simulink model "Bebop10_from_exp"  (R2018a)
settings: Solver=VariableStepAuto  StartTime=0.0  StopTime=100  FixedStep=0.0025  MaxStep=1  MinStep=0.005  RelTol=10  AbsTol=10
values from neighbouring files (symbols this model uses):
  flightplan = [dist,0,height,deg2rad(090) ... (first row only)    [compare_cubic_spline_1.m]    (also in initialize_race_realtime.m = flightplan - [0.5*min(flightplan(:,1:2))+0.5*max(flightplan(; initialize_race_realtime_backup_cubic.m; plot_sim.m = [ 4.348, -0.278, height, deg2rad(  0); test_b_spline.m)
  FOV = 1.05    [initialize_race_realtime_backup_cubic.m]
  g = 9.81    [initialize_race_no_realtime.m]    (also in initialize_race_realtime.m; initialize_race_realtime_backup_cubic.m; moving_average_rls_own.m = P(i-1)*meas*(lambda+meas*P(i-1)*meas)^-1)
  gate_size = 1.4    [initialize_race_realtime.m]    (also in initialize_race_realtime_backup_cubic.m)
  gates = sim_gates(:,:,1)    [eval_sim.m]    (also in initialize_race_realtime.m = flightplan + pert; initialize_race_realtime_backup_cubic.m = [dist,0,height,deg2rad(110); plot_sim.m)
  HFOV = VFOV*resolution(1)/resolution(2)    [initialize_race_realtime.m]
  I = [1 0 0 ... (first row only)    [Bebop_sim_init.m]    (also in initialize_race_no_realtime.m; initialize_race_realtime.m; initialize_race_realtime_backup_cubic.m; moving_averge_rls_download.m = ones(1,N))
  m = 0.68    [calc_plot_spline.m]    (also in calc_spline.m; compare_cubic_spline_1.m = vpasolve(e,r); compare_cubic_spline_2.m = r/3*(-sin(dp)+sqrt(sin(dp)^2-6*cos(dp)+6)); initialize_race_no_realtime.m = 2)
  mass = 2    [Bebop_sim_init.m]    (also in initialize_race_realtime.m = 0.5)
  max_rot_Z = (90)*pi/180    (= 1.57079632679)    [Bebop_sim_init.m]    (also in initialize_race_no_realtime.m = 1.0471975512; initialize_race_realtime.m = 3.14159265359; initialize_race_realtime_backup_cubic.m; run_batch1.m = list_agility(idx_agility)*max_rot_Z)
  max_theta_X = (40)*pi/180    (= 0.698131700798)    [Bebop_sim_init.m]    (also in initialize_race_no_realtime.m = 0.13962634016; initialize_race_realtime.m = 0.418879020479; initialize_race_realtime_backup_cubic.m = 1.308996939; run_batch1.m = list_agility(idx_agility)*max_theta_X)
  max_theta_Y = (40)*pi/180    (= 0.698131700798)    [Bebop_sim_init.m]    (also in initialize_race_no_realtime.m = 0.13962634016; initialize_race_realtime.m = 0.418879020479; initialize_race_realtime_backup_cubic.m = 1.308996939; run_batch1.m = list_agility(idx_agility)*max_theta_Y)
  max_v_Z = .5    (= 0.5)    [Bebop_sim_init.m]    (also in initialize_race_no_realtime.m = 1; initialize_race_realtime.m = 6; initialize_race_realtime_backup_cubic.m = 3; run_batch1.m = list_agility(idx_agility)*max_v_Z)
  max_vel = 2.0    (= 2)    [initialize_race_realtime.m]    (also in initialize_race_realtime_backup_cubic.m = 1.5; run_batch1.m = list_speed(idx_speed); run_batch2.m = list_speed(idx_speed); run_batch3.m = list_speed(idx_speed))
  resolution = 0.5*[1280 720]    [initialize_race_realtime.m]
  spline_init = [P0;P1;P2;P3]    [initialize_race_realtime.m]
  std_dev_eul = 0.25*deg2rad(0.8)*ones(1,3)    [initialize_race_realtime.m]    (also in run_batch1.m = list_sensor_eul(idx_sensor)*dist*ones(1,3); run_batch2.m = list_sensor_eul(idx_sensor)*dist*ones(1,3); run_batch3.m = list_sensor_eul(idx_sensor)*dist*ones(1,3); run_batch4.m = list_sensor_eul(idx_sensor)*dist*ones(1,3))
  std_dev_F = 0.1*max_force*ones(1,3)    [initialize_race_realtime.m]    (also in run_batch1.m = list_actuator(idx_actuator)*max_force*ones(1,3); run_batch2.m = list_actuator(idx_actuator)*max_force*ones(1,3); run_batch3.m = list_actuator(idx_sensor)*max_force*ones(1,3); run_batch4.m = list_actuator(idx_sensor)*max_force*ones(1,3))
  std_dev_M = 0.1*max_moment*[0, 0, 1]    [initialize_race_realtime.m]    (also in run_batch1.m = list_actuator(idx_actuator)*max_moment*[0, 0, 1]; run_batch2.m = list_actuator(idx_actuator)*max_moment*[0, 0, 1]; run_batch3.m = list_actuator(idx_sensor)*max_moment*[0, 0, 1]; run_batch4.m = list_actuator(idx_sensor)*max_moment*[0, 0, 1])
  std_dev_vel = 0.06*ones(1,3)    [initialize_race_realtime.m]    (also in run_batch1.m = list_sensor(idx_sensor)*dist*ones(1,3); run_batch2.m = list_sensor(idx_sensor)*dist*ones(1,3); run_batch3.m = list_sensor(idx_sensor)*dist*ones(1,3); run_batch4.m = list_sensor(idx_sensor)*dist*ones(1,3))
  std_dev_xyz = 0.06*ones(1,3)    [initialize_race_realtime.m]    (also in run_batch1.m = list_sensor(idx_sensor)*dist*ones(1,3); run_batch2.m = list_sensor(idx_sensor)*dist*ones(1,3); run_batch3.m = list_sensor(idx_sensor)*dist*ones(1,3); run_batch4.m = list_sensor(idx_sensor)*dist*ones(1,3))
  two_std_dev_init = [1,1,0.5,deg2rad(30)]    [initialize_race_realtime.m]
  two_std_dev_thres = 0.3    [initialize_race_realtime.m]
  VFOV = 1.05    [initialize_race_realtime.m]
undefined symbols (not defined in the file or in its folder): gray, Rec, SDTV
libraries: sharedtransform x13, visiontextngfix x5, aerolibactuator x4, simulink x3, aerolibutil x2, visionconversions x2, shared6dof x1, vrlib x1, visionanalysis x1, visionstatistics x1, visiontransforms x1
(part 1 of 3)
settings Model: Creator=vinni  LastModifiedBy=lenny
settings SolverCC: MaxConsecutiveMinStep=99999  ShapePreserveControl=EnableAll  ZeroCrossAlgorithm=Adaptive
settings DebuggingCC: RTPrefix=warning  StringTruncationChecking=warning  WriteAfterWriteMsg=EnableAllAsError  MaxConsecutiveZCsMsg=warning  MultiTaskDSMMsg=warning  MultiTaskCondExecSysMsg=warning  MultiTaskRateTransMsg=warning  ParameterDowncastMsg=warning  ParameterOverflowMsg=warning  ParameterUnderflowMsg=warning  InvalidFcnCallConnMsg=warning  FcnCallInpInsideContextMsg=warning  UniqueDataStoreMsg=warning  ModelReferenceExtraNoncontSigs=warning  NonBusSignalsTreatedAsBus=error
settings HardwareCC: ProdBitPerLong=64  ProdHWDeviceType=Intel->x86-64 (Linux 64)

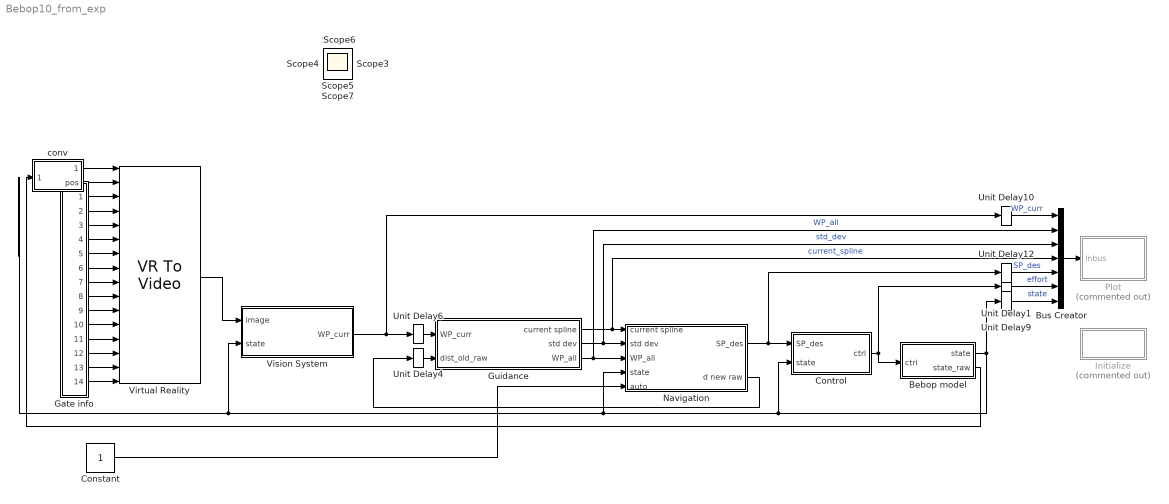
== system Bebop10_from_exp ==
  Bebop model : Subsystem
  Bus Creator : BusCreator  Inputs=7  OutDataTypeStr=Bus: PlotBus  NonVirtualBus=on
  Constant : Constant
  Control : Subsystem
  Gate info : Subsystem
  Guidance : Subsystem
  Initialize : Subsystem  Commented=on  TreatAsAtomicUnit=on
  Navigation : Subsystem
  Plot : MATLAB Function  Commented=on  TreatAsAtomicUnit=on
  Unit Delay{1,4,6,9..10,12} (6 alike) : UnitDelay  SampleTime=-1
  Virtual Reality : vrlib/VR To Video  InstantiateOnLoad=on  SampleTime=0.200  ViewEnable=on  RemoteChange=off  RemoteView=off  FieldsWritten=drone.orientation.4.1.1.double#drone.position.3.1.1.double#G1.rotation.4.1.1.double#G1.translation.3.1.1.double#G2.rotation.4.1.1.double#G2.translation.3.1.1.double#G3.rotation.4.1.1.double#G3.translation.3.1.1.double#G4.rotation.4.1.1.double#G4.translation.3.1.1.double#G5.rotation.4.1.1.double#G5.translation.3.1.1.double#G6.rotation.4.1.1.double#G6.translation.3.1.1.double#G7.rotation.4.1.1.double#G7.translation.3.1.1.double  WorldFileName=race_course.wrl  AutoView=off  VideoDimensions=0.5*[720 1280]  AllowVariableSize=off  FigureProperties="{'Position', 'Name', 'Viewpoint', 'CameraBound', 'CameraDirection', 'CameraPosition', 'CameraUpVector', 'ZoomFactor', 'Antialiasing', 'Headlight', 'Lighting', 'NavPanel', 'Sound', 'StatusBar', 'Stereo3D', 'Stereo3DCameraOffset', 'Stereo3DHIT', 'ToolBar', 'Textures', 'Transparency', 'Triad', 'Wireframe', 'NavZones', 'NavMode', 'NavSpeed', 'CaptureFileFormat', 'CaptureFileName', 'Record2DCompressMethod', 'Record2DCompressQuality', 'Record2D', 'Record2DFileName', 'Record2DFPS'; [3.0000000000000000e+01   6.0000000000000000e+01   6.4000000000000000e+02   3.6000000000000000e+02], '', '_untitled_1', 'on', [0.0000000000000000e+00   0.0000000000000000e+00  -1.0000000000000000e+00], [0.0000000000000000e+00   0.0000000000000000e+00   0.0000000000000000e+00], [0.0000000000000000e+00   1.0000000000000000e+00   0.0000000000000000e+00], [1.0000000000000000e+00], 'off', 'on', 'on', 'none', 'on', 'off', 'off', [1.0000000149011612e-01], [0.0000000000000000e+00], 'off', 'on', 'on', 'none', 'off', 'off', 'fly', 'normal', 'tif', '%f_anim_%n.tif', 'auto', [7.5000000000000000e+01], 'off', '***video***', 'auto'}"
      settings: SourceProductName=Simulink 3D Animation  SourceProductBaseCode=VR
  Vision System : Subsystem
  conv : Subsystem
  Scope{,1..7} (8 alike) : Scope
  wires:
  Vision System/1(WP_curr) -> Unit Delay10/1, Unit Delay6/1
  Control/1(ctrl) -> Bebop model/1(ctrl), Unit Delay1/1
  Unit Delay6/1 -> Guidance/1(WP_curr)
  Unit Delay4/1 -> Guidance/2(dist_old_raw)
  Navigation/1(SP_des) -> Unit Delay12/1, Control/1(SP_des)
  Navigation/2(d new raw) -> Unit Delay4/1
  Bus Creator/1 -> Plot/1(inbus)
  Guidance/3(WP_all) -> Navigation/3(WP_all), Bus Creator/2  "WP_all"
  Guidance/2(std dev) -> Navigation/2(std dev), Bus Creator/3  "std_dev"
  Unit Delay9/1 -> Bus Creator/7  "state"
  Unit Delay10/1 -> Bus Creator/1  "WP_curr"
  Unit Delay12/1 -> Bus Creator/5  "SP_des"
  Guidance/1(current spline) -> Navigation/1(current spline), Bus Creator/4  "current_spline"
  Unit Delay1/1 -> Bus Creator/6  "effort"
  Virtual Reality/1 -> Vision System/1(image)
  Constant/1 -> Navigation/5(auto)
  Bebop model/1(state) -> Control/2(state), Navigation/4(state), Vision System/2(state), Unit Delay9/1
  conv/1(axang) -> Virtual Reality/1
  conv/2(pos) -> Virtual Reality/2
  Gate info/1(O1) -> Virtual Reality/3
  Gate info/2(P1) -> Virtual Reality/4
  Gate info/3(O2) -> Virtual Reality/5
  Gate info/4(P2) -> Virtual Reality/6
  Gate info/5(O3) -> Virtual Reality/7
  Gate info/6(P3) -> Virtual Reality/8
  Gate info/7(O4) -> Virtual Reality/9
  Gate info/8(P4) -> Virtual Reality/10
  Gate info/9(O5) -> Virtual Reality/11
  Gate info/10(P5) -> Virtual Reality/12
  Gate info/11(O6) -> Virtual Reality/13
  Gate info/12(P6) -> Virtual Reality/14
  Gate info/13(O7) -> Virtual Reality/15
  Gate info/14(P7) -> Virtual Reality/16
  Bebop model/2(state_raw) -> conv/1(state)

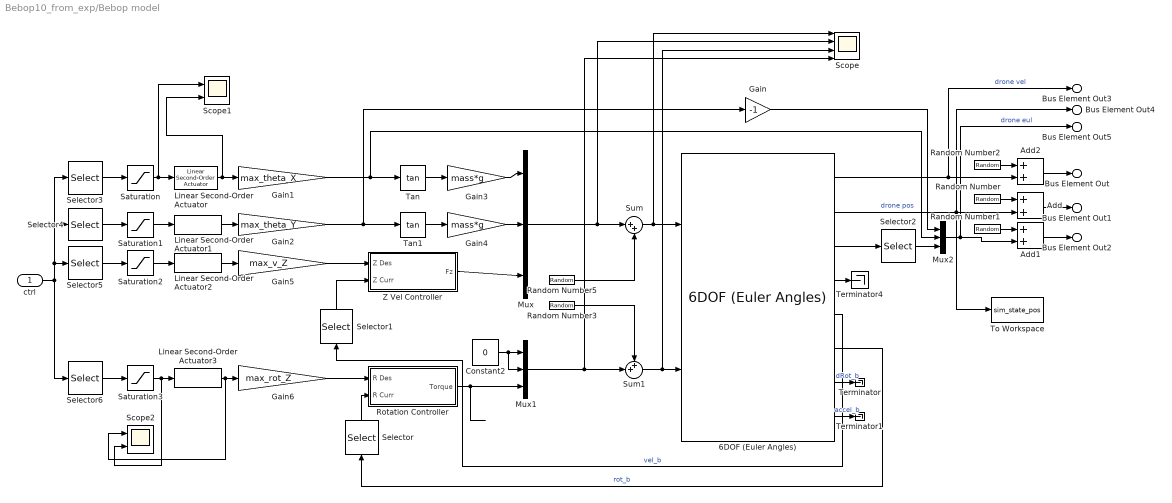
== system Bebop10_from_exp/Bebop model ==
  ctrl : Inport
  6DOF (Euler Angles) : shared6dof/6DOF (Euler Angles)  units=Metric (MKS)  mtype=Fixed  rep=Euler Angles  xme_0=Initial_pos  Vm_0=Initial_vel_b  eul_0=Initial_ori  pm_0=[0 0 0]  mass_0=mass  mass_e=0.5  mass_f=2.0  inertia=I  inertia_e=eye(3)  inertia_f=2*eye(3)  k_quat=1.0  vre_flag=on  abi_flag=off  aMode=0
      settings: SourceProductBaseCode=AE
  Add : Sum
  Add1 : Sum
  Add2 : Sum
  Constant2 : Constant  Value=0
  Gain : Gain  Gain=-1
  Gain1 : Gain  Gain=max_theta_X
  Gain2 : Gain  Gain=max_theta_Y
  Gain3 : Gain  Gain=mass*g
  Gain4 : Gain  Gain=mass*g
  Gain5 : Gain  Gain=max_v_Z
  Gain6 : Gain  Gain=max_rot_Z
  Linear Second-Order Actuator : aerolibactuator/Linear Second-Order Actuator  wn_fin=20  z_fin=3  fin_act_0=0  fin_act_vel=0
      settings: SourceProductName=Aerospace Blockset  SourceProductBaseCode=AE
  Linear Second-Order Actuator1 : aerolibactuator/Linear Second-Order Actuator  wn_fin=20  z_fin=3  fin_act_0=0  fin_act_vel=0
      settings: SourceProductName=Aerospace Blockset  SourceProductBaseCode=AE
  Linear Second-Order Actuator2 : aerolibactuator/Linear Second-Order Actuator  wn_fin=20  z_fin=1  fin_act_0=0  fin_act_vel=0
      settings: SourceProductName=Aerospace Blockset  SourceProductBaseCode=AE
  Linear Second-Order Actuator3 : aerolibactuator/Linear Second-Order Actuator  wn_fin=20  z_fin=1  fin_act_0=0  fin_act_vel=0
      settings: SourceProductName=Aerospace Blockset  SourceProductBaseCode=AE
  Mux : Mux  Inputs=3
  Mux1 : Mux  Inputs=3
  Mux2 : Mux  Inputs=3
  Random Number : RandomNumber  Mean=0*ones(1,3)  Variance=std_dev_xyz.^2.*ones(1,3)  Seed=[4,5,6]  SampleTime=0.1
  Random Number1 : RandomNumber  Mean=0*ones(1,3)  Variance=std_dev_eul.^2.*ones(1,3)  Seed=[7,8,9]  SampleTime=0.1
  Random Number2 : RandomNumber  Mean=0*ones(1,3)  Variance=std_dev_vel.^2.*ones(1,3)  Seed=[1,2,3]  SampleTime=0.1
  Random Number3 : RandomNumber  Mean=0*ones(1,3)  Variance=std_dev_M.^2.*ones(1,3)  Seed=[13,14,15]  SampleTime=0.1
  Random Number5 : RandomNumber  Mean=0*ones(1,3)  Variance=std_dev_F.^2.*ones(1,3)  Seed=[10,11,12]  SampleTime=0.1
  Rotation Controller : Subsystem
  Saturation{,1..3} (4 alike) : Saturate  UpperLimit=1  LowerLimit=-1
  Scope : Scope  NumInputPorts=4
  Scope1 : Scope  NumInputPorts=2
  Scope2 : Scope  NumInputPorts=2
  Selector : Selector  InputPortWidth=3  IndexOptions=Index vector (dialog)  Indices=3  OutputSizes=1
  Selector1 : Selector  InputPortWidth=3  IndexOptions=Index vector (dialog)  Indices=3  OutputSizes=1
  Selector2 : Selector  InputPortWidth=3  IndexOptions=Index vector (dialog)  Indices=3  OutputSizes=1
  Selector3 : Selector  IndexMode=Zero-based  InputPortWidth=4  IndexOptions=Index vector (dialog)  Indices=0  OutputSizes=1
  Selector4 : Selector  IndexMode=Zero-based  InputPortWidth=4  IndexOptions=Index vector (dialog)  Indices=1  OutputSizes=1
  Selector5 : Selector  IndexMode=Zero-based  InputPortWidth=4  IndexOptions=Index vector (dialog)  Indices=2  OutputSizes=1
  Selector6 : Selector  IndexMode=Zero-based  InputPortWidth=4  IndexOptions=Index vector (dialog)  Indices=3  OutputSizes=1
  Sum : Sum  Inputs=|++
  Sum1 : Sum  Inputs=++|
  Tan : Trigonometry  Operator=tan
  Tan1 : Trigonometry  Operator=tan
  Terminator : Terminator
  Terminator1 : Terminator
  Terminator4 : Terminator
  To Workspace : ToWorkspace  VariableName=sim_state_pos  SaveFormat=Timeseries  SampleTime=-1
  Z Vel Controller : Subsystem
  Bus Element Out : Outport  PortName=state  Element=vel
  Bus Element Out1 : Outport  PortName=state  Element=pos
  Bus Element Out2 : Outport  PortName=state  Element=eul
  Bus Element Out3 : Outport  Port=2  PortName=state_raw  Element=vel
  Bus Element Out4 : Outport  Port=2  PortName=state_raw  Element=pos
  Bus Element Out5 : Outport  Port=2  PortName=state_raw  Element=eul
  wires:
  6DOF (Euler Angles)/5 -> Selector1/1  "vel_b"
  Saturation/1 -> Scope1/1, Linear Second-Order Actuator/1
  Tan1/1 -> Gain4/1
  Selector6/1 -> Saturation3/1
  Linear Second-Order Actuator1/1 -> Gain2/1
  Z Vel Controller/1(Fz) -> Mux/3
  6DOF (Euler Angles)/1 -> Bus Element Out3/1, Add2/2  "drone vel"
  Rotation Controller/1(Torque) -> Mux1/3
  Selector/1 -> Rotation Controller/2(R Curr)
  Selector1/1 -> Z Vel Controller/2(Z Curr)
  Gain3/1 -> Mux/1
  Saturation1/1 -> Linear Second-Order Actuator1/1
  6DOF (Euler Angles)/3 -> Selector2/1
  Selector5/1 -> Saturation2/1
  Gain1/1 -> Mux2/2, Tan/1
  Mux/1 -> Scope/2, Sum/1
  Gain5/1 -> Z Vel Controller/1(Z Des)
  Selector4/1 -> Saturation1/1
  Tan/1 -> Gain3/1
  Gain/1 -> Mux2/1
  6DOF (Euler Angles)/4 -> Terminator4/1
  Constant2/1 -> Mux1/2, Mux1/1
  Saturation2/1 -> Linear Second-Order Actuator2/1
  Gain2/1 -> Tan1/1, Gain/1
  Saturation3/1 -> Scope2/2, Linear Second-Order Actuator3/1
  Linear Second-Order Actuator/1 -> Scope1/2, Gain1/1
  Mux1/1 -> Scope/4, Sum1/2
  Gain6/1 -> Rotation Controller/1(R Des)
  Gain4/1 -> Mux/2
  Selector3/1 -> Saturation/1
  6DOF (Euler Angles)/6 -> Selector/1  "rot_b"
  Selector2/1 -> Mux2/3
  6DOF (Euler Angles)/2 -> Bus Element Out4/1, To Workspace/1, Add/2  "drone pos"
  Mux2/1 -> Bus Element Out5/1, Add1/2  "drone eul"
  ctrl/1 -> Selector5/1, Selector4/1, Selector3/1, Selector6/1
  6DOF (Euler Angles)/7 -> Terminator/1  "dRot_b"
  6DOF (Euler Angles)/8 -> Terminator1/1  "accel_b"
  Random Number/1 -> Add/1
  Add/1 -> Bus Element Out1/1
  Random Number2/1 -> Add2/1
  Random Number1/1 -> Add1/1
  Add2/1 -> Bus Element Out/1
  Add1/1 -> Bus Element Out2/1
  Linear Second-Order Actuator2/1 -> Gain5/1
  Linear Second-Order Actuator3/1 -> Scope2/1, Gain6/1
  Sum/1 -> Scope/1, 6DOF (Euler Angles)/1
  Random Number5/1 -> Sum/2
  Random Number3/1 -> Sum1/1
  Sum1/1 -> Scope/3, 6DOF (Euler Angles)/2

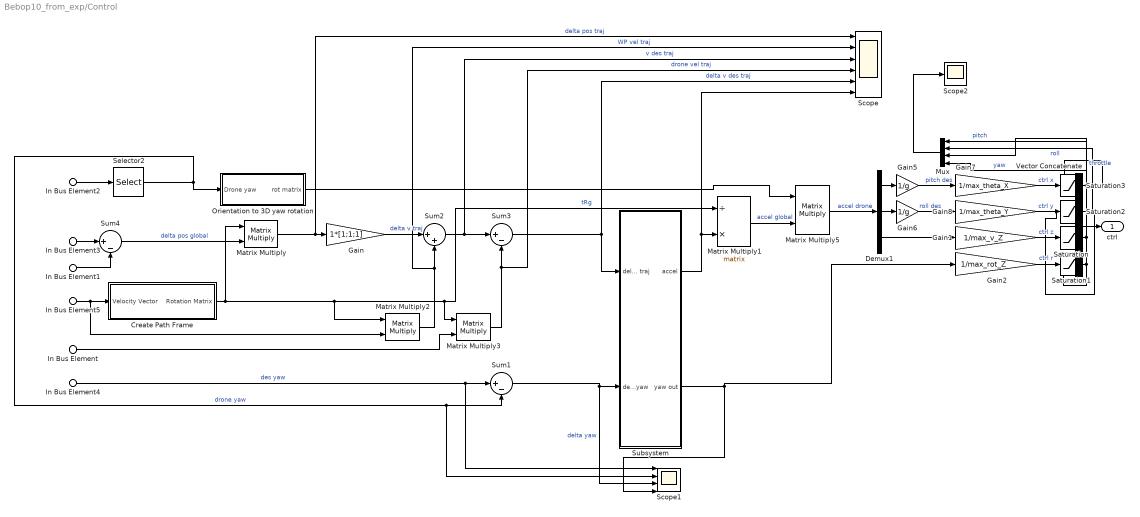
== system Bebop10_from_exp/Control ==
  In Bus Element5 : Inport  PortName=SP_des  Element=vel
  In Bus Element3 : Inport  PortName=SP_des  Element=pos
  In Bus Element4 : Inport  PortName=SP_des  Element=yaw
  In Bus Element : Inport  Port=2  PortName=state  Element=vel
  In Bus Element1 : Inport  Port=2  PortName=state  Element=pos
  In Bus Element2 : Inport  Port=2  PortName=state  Element=eul
  Create Path Frame : Subsystem
  Demux1 : Demux  Outputs=3
  Gain : Gain  Gain=1*[1;1;1]
  Gain1 : Gain  Gain=1/max_v_Z
  Gain2 : Gain  Gain=1/max_rot_Z
  Gain5 : Gain  Gain=1/g
  Gain6 : Gain  Gain=1/g
  Gain7 : Gain  Gain=1/max_theta_X
  Gain8 : Gain  Gain=1/max_theta_Y
  Matrix Multiply{,2..3,5} (4 alike) : Product  Inputs=**  Multiplication=Matrix(*)
  Matrix Multiply1 : Product  Inputs=/*  Multiplication=Matrix(*)
  Mux : Mux
  Orientation to 3D yaw rotation : Subsystem
  Saturation{,1..3} (4 alike) : Saturate  UpperLimit=1  LowerLimit=-1
  Scope : Scope  NumInputPorts=6
  Scope1 : Scope  NumInputPorts=4
  Scope2 : Scope
  Selector2 : Selector  IndexMode=Zero-based  InputPortWidth=3  IndexOptions=Index vector (dialog)  Indices=2  OutputSizes=1
  Subsystem : Subsystem
  Sum1 : Sum  Inputs=|+-
  Sum2 : Sum  Inputs=|++
  Sum3 : Sum  Inputs=|+-
  Sum4 : Sum  Inputs=|+-
  Vector Concatenate : Concatenate  NumInputs=4
  ctrl : Outport
  wires:
  Saturation1/1 -> Vector Concatenate/4, Mux/4  "yaw"
  Saturation3/1 -> Vector Concatenate/1, Mux/1  "pitch"
  Saturation2/1 -> Mux/2, Vector Concatenate/2  "roll"
  Saturation/1 -> Vector Concatenate/3, Mux/3  "throttle"
  In Bus Element4/1 -> Scope1/1, Sum1/1  "des yaw"
  In Bus Element5/1 -> Matrix Multiply2/2, Create Path Frame/1(Velocity Vector)
  Selector2/1 -> Scope1/2, Sum1/2, Orientation to 3D yaw rotation/1(Drone yaw)  "drone yaw"
  Gain7/1 -> Saturation3/1  "ctrl x"
  Demux1/3 -> Gain1/1
  Demux1/2 -> Gain6/1
  Mux/1 -> Scope2/1
  Gain6/1 -> Gain8/1  "roll des"
  Sum3/1 -> Scope/5, Subsystem/1(delta v des traj)  "delta v des traj"
  Matrix Multiply2/1 -> Scope/2, Sum2/2  "WP vel traj"
  Sum4/1 -> Matrix Multiply/2  "delta pos global"
  Matrix Multiply3/1 -> Scope/4, Sum3/2  "drone vel traj"
  Demux1/1 -> Gain5/1
  Gain1/1 -> Saturation/1  "ctrl z"
  Matrix Multiply/1 -> Scope/1, Gain/1  "delta pos traj"
  Gain5/1 -> Gain7/1  "pitch des"
  Matrix Multiply5/1 -> Demux1/1  "accel drone"
  Orientation to 3D yaw rotation/1(rot matrix) -> Matrix Multiply5/1
  Gain8/1 -> Saturation2/1  "ctrl y"
  In Bus Element1/1 -> Sum4/2
  Create Path Frame/1(Rotation Matrix) -> Matrix Multiply/1, Matrix Multiply2/1, Matrix Multiply1/1, Matrix Multiply3/1  "tRg"
  Gain2/1 -> Saturation1/1  "ctrl r"
  In Bus Element/1 -> Matrix Multiply3/2
  Gain/1 -> Sum2/1  "delta v traj"
  Sum2/1 -> Scope/3, Sum3/1  "v des traj"
  Matrix Multiply1/1 -> Matrix Multiply5/2  "accel global"
  Sum1/1 -> Scope1/3, Subsystem/2(delta yaw)  "delta yaw"
  In Bus Element2/1 -> Selector2/1
  Vector Concatenate/1 -> ctrl/1
  Subsystem/1(accel) -> Scope/6, Matrix Multiply1/2
  Subsystem/2(yaw out) -> Gain2/1, Scope1/4
  In Bus Element3/1 -> Sum4/1

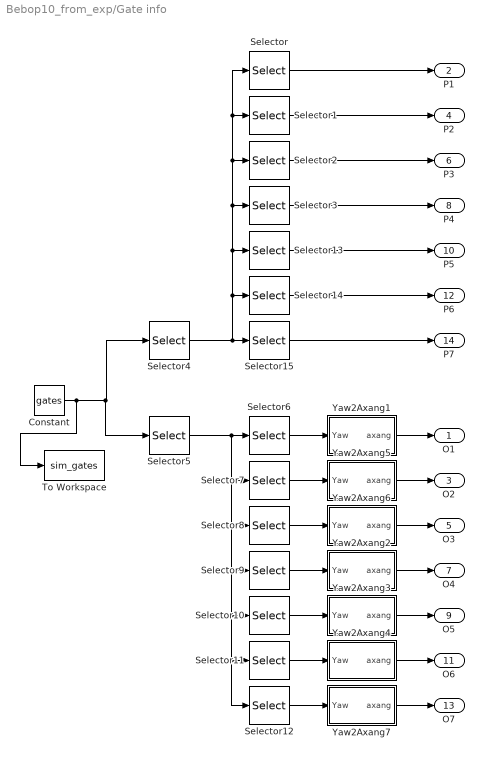
== system Bebop10_from_exp/Gate info ==
  Constant : Constant  Value=gates
  Selector : Selector  NumberOfDimensions=2  IndexMode=Zero-based  InputPortWidth=3  IndexOptions=Index vector (dialog),Select all  Indices=0,1  OutputSizes=1,1
  Selector1 : Selector  NumberOfDimensions=2  IndexMode=Zero-based  InputPortWidth=3  IndexOptions=Index vector (dialog),Select all  Indices=1,1  OutputSizes=1,1
  Selector10 : Selector  NumberOfDimensions=2  IndexMode=Zero-based  InputPortWidth=3  IndexOptions=Index vector (dialog),Select all  Indices=4,1  OutputSizes=1,1
  Selector11 : Selector  NumberOfDimensions=2  IndexMode=Zero-based  InputPortWidth=3  IndexOptions=Index vector (dialog),Select all  Indices=5,1  OutputSizes=1,1
  Selector12 : Selector  NumberOfDimensions=2  IndexMode=Zero-based  InputPortWidth=3  IndexOptions=Index vector (dialog),Select all  Indices=6,1  OutputSizes=1,1
  Selector13 : Selector  NumberOfDimensions=2  IndexMode=Zero-based  InputPortWidth=3  IndexOptions=Index vector (dialog),Select all  Indices=4,1  OutputSizes=1,1
  Selector14 : Selector  NumberOfDimensions=2  IndexMode=Zero-based  InputPortWidth=3  IndexOptions=Index vector (dialog),Select all  Indices=5,1  OutputSizes=1,1
  Selector15 : Selector  NumberOfDimensions=2  IndexMode=Zero-based  InputPortWidth=3  IndexOptions=Index vector (dialog),Select all  Indices=6,1  OutputSizes=1,1
  Selector2 : Selector  NumberOfDimensions=2  IndexMode=Zero-based  InputPortWidth=3  IndexOptions=Index vector (dialog),Select all  Indices=2,1  OutputSizes=1,1
  Selector3 : Selector  NumberOfDimensions=2  IndexMode=Zero-based  InputPortWidth=3  IndexOptions=Index vector (dialog),Select all  Indices=3,1  OutputSizes=1,1
  Selector4 : Selector  NumberOfDimensions=2  IndexMode=Zero-based  InputPortWidth=3  IndexOptions=Select all,Index vector (dialog)  Indices=4,[0 1 2]  OutputSizes=1,1
  Selector5 : Selector  NumberOfDimensions=2  IndexMode=Zero-based  InputPortWidth=3  IndexOptions=Select all,Index vector (dialog)  Indices=4,3  OutputSizes=1,1
  Selector6 : Selector  NumberOfDimensions=2  IndexMode=Zero-based  InputPortWidth=3  IndexOptions=Index vector (dialog),Select all  Indices=0,1  OutputSizes=1,1
  Selector7 : Selector  NumberOfDimensions=2  IndexMode=Zero-based  InputPortWidth=3  IndexOptions=Index vector (dialog),Select all  Indices=1,1  OutputSizes=1,1
  Selector8 : Selector  NumberOfDimensions=2  IndexMode=Zero-based  InputPortWidth=3  IndexOptions=Index vector (dialog),Select all  Indices=2,1  OutputSizes=1,1
  Selector9 : Selector  NumberOfDimensions=2  IndexMode=Zero-based  InputPortWidth=3  IndexOptions=Index vector (dialog),Select all  Indices=3,1  OutputSizes=1,1
  To Workspace : ToWorkspace  VariableName=sim_gates  SaveFormat=Timeseries  SampleTime=-1
  Yaw2Axang1 : Subsystem
  Yaw2Axang2 : Subsystem
  Yaw2Axang3 : Subsystem
  Yaw2Axang4 : Subsystem
  Yaw2Axang5 : Subsystem
  Yaw2Axang6 : Subsystem
  Yaw2Axang7 : Subsystem
  O1 : Outport
  P1 : Outport  Port=2
  O2 : Outport  Port=3
  P2 : Outport  Port=4
  O3 : Outport  Port=5
  P3 : Outport  Port=6
  O4 : Outport  Port=7
  P4 : Outport  Port=8
  O5 : Outport  Port=9
  P5 : Outport  Port=10
  O6 : Outport  Port=11
  P6 : Outport  Port=12
  O7 : Outport  Port=13
  P7 : Outport  Port=14
  wires:
  Selector/1 -> P1/1
  Selector3/1 -> P4/1
  Selector2/1 -> P3/1
  Selector4/1 -> Selector15/1, Selector14/1, Selector13/1, Selector1/1, Selector/1, Selector2/1, Selector3/1
  Selector1/1 -> P2/1
  Constant/1 -> To Workspace/1, Selector5/1, Selector4/1
  Selector5/1 -> Selector12/1, Selector11/1, Selector10/1, Selector9/1, Selector8/1, Selector7/1, Selector6/1
  Selector6/1 -> Yaw2Axang1/1(Yaw)
  Selector7/1 -> Yaw2Axang5/1(Yaw)
  Selector8/1 -> Yaw2Axang6/1(Yaw)
  Selector9/1 -> Yaw2Axang2/1(Yaw)
  Yaw2Axang1/1(axang) -> O1/1
  Yaw2Axang5/1(axang) -> O2/1
  Yaw2Axang6/1(axang) -> O3/1
  Yaw2Axang2/1(axang) -> O4/1
  Yaw2Axang3/1(axang) -> O5/1
  Selector10/1 -> Yaw2Axang3/1(Yaw)
  Yaw2Axang4/1(axang) -> O6/1
  Selector11/1 -> Yaw2Axang4/1(Yaw)
  Yaw2Axang7/1(axang) -> O7/1
  Selector12/1 -> Yaw2Axang7/1(Yaw)
  Selector13/1 -> P5/1
  Selector14/1 -> P6/1
  Selector15/1 -> P7/1

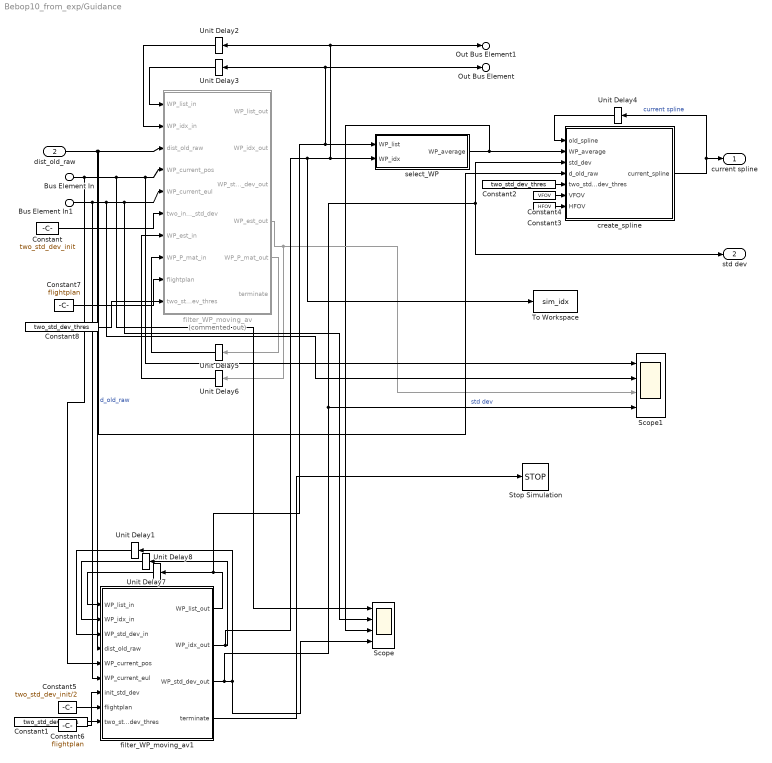
== system Bebop10_from_exp/Guidance ==
  Bus Element In1 : Inport  PortName=WP_curr  Element=eul
  Bus Element In : Inport  PortName=WP_curr  Element=pos
  dist_old_raw : Inport  Port=2
  Constant : Constant  Value=two_std_dev_init
  Constant1 : Constant  Value=two_std_dev_thres
  Constant2 : Constant  Value=two_std_dev_thres
  Constant3 : Constant  Value=HFOV
  Constant4 : Constant  Value=VFOV
  Constant5 : Constant  Value=two_std_dev_init/2
  Constant6 : Constant  Value=flightplan
  Constant7 : Constant  Value=flightplan
  Constant8 : Constant  Value=two_std_dev_thres
  Scope : Scope  NumInputPorts=4
  Scope1 : Scope  NumInputPorts=4
  Stop Simulation : Stop
  To Workspace : ToWorkspace  VariableName=sim_idx  SaveFormat=Timeseries  SampleTime=-1
  Unit Delay1 : UnitDelay  InitialCondition=two_std_dev_init/2  SampleTime=-1
  Unit Delay2 : UnitDelay  SampleTime=-1
  Unit Delay3 : UnitDelay  InitialCondition=flightplan  SampleTime=-1
  Unit Delay4 : UnitDelay  InitialCondition=spline_init  SampleTime=-1
  Unit Delay5 : UnitDelay  InitialCondition=ones(4,4)  SampleTime=-1
  Unit Delay6 : UnitDelay  InitialCondition=ones(1,4)  SampleTime=-1
  Unit Delay7 : UnitDelay  SampleTime=-1
  Unit Delay8 : UnitDelay  InitialCondition=flightplan  SampleTime=-1
  create_spline : MATLAB Function  TreatAsAtomicUnit=on
  filter_WP_moving_av : MATLAB Function  Commented=on  TreatAsAtomicUnit=on
  filter_WP_moving_av1 : MATLAB Function  TreatAsAtomicUnit=on
  select_WP : MATLAB Function  TreatAsAtomicUnit=on
  current spline : Outport
  std dev : Outport  Port=2
  Out Bus Element : Outport  Port=3  PortName=WP_all  Element=list
  Out Bus Element1 : Outport  Port=3  PortName=WP_all  Element=idx
  wires:
  create_spline/1(current_spline) -> Unit Delay4/1, current spline/1  "current spline"
  select_WP/1(WP_average) -> Scope/3, create_spline/2(WP_average)
  Unit Delay3/1 -> filter_WP_moving_av/1(WP_list_in)
  Unit Delay2/1 -> filter_WP_moving_av/2(WP_idx_in)
  Constant/1 -> filter_WP_moving_av/6(two_init_std_dev)
  Unit Delay4/1 -> create_spline/1(old_spline)
  filter_WP_moving_av/4(WP_est_out) -> Unit Delay6/1, Scope1/3
  filter_WP_moving_av/5(WP_P_mat_out) -> Unit Delay5/1
  Unit Delay5/1 -> filter_WP_moving_av/8(WP_P_mat_in)
  Unit Delay6/1 -> filter_WP_moving_av/7(WP_est_in)
  Constant2/1 -> create_spline/5(two_std_dev_thres)
  Constant3/1 -> create_spline/7(HFOV)
  Constant4/1 -> create_spline/6(VFOV)
  dist_old_raw/1 -> filter_WP_moving_av/3(dist_old_raw), create_spline/4(d_old_raw), filter_WP_moving_av1/4(dist_old_raw)  "d_old_raw"
  Unit Delay7/1 -> filter_WP_moving_av1/2(WP_idx_in)
  Bus Element In1/1 -> filter_WP_moving_av1/6(WP_current_eul), Scope1/2, Scope/2, filter_WP_moving_av/5(WP_current_eul)
  Bus Element In/1 -> filter_WP_moving_av1/5(WP_current_pos), Scope/1, Scope1/1, filter_WP_moving_av/4(WP_current_pos)
  Constant5/1 -> filter_WP_moving_av1/7(init_std_dev)
  Unit Delay1/1 -> filter_WP_moving_av1/3(WP_std_dev_in)
  Unit Delay8/1 -> filter_WP_moving_av1/1(WP_list_in)
  Constant6/1 -> filter_WP_moving_av1/8(flightplan)
  filter_WP_moving_av1/3(WP_std_dev_out) -> std dev/1, create_spline/3(std_dev), Scope1/4, Scope/4, Unit Delay1/1  "std dev"
  Constant7/1 -> filter_WP_moving_av/9(flightplan)
  Constant1/1 -> filter_WP_moving_av1/9(two_std_dev_thres)
  filter_WP_moving_av1/1(WP_list_out) -> Out Bus Element/1, Unit Delay3/1, select_WP/1(WP_list), Unit Delay8/1
  filter_WP_moving_av1/2(WP_idx_out) -> To Workspace/1, Out Bus Element1/1, Unit Delay2/1, select_WP/2(WP_idx), Unit Delay7/1
  Constant8/1 -> filter_WP_moving_av/10(two_std_dev_thres)
  filter_WP_moving_av1/4(terminate) -> Stop Simulation/1

== system Bebop10_from_exp/Initialize ==
  Constant : Constant  Value=gates
  Event Listener : EventListener  DisableCoverage=on  EventName=reset
  reset_plot : MATLAB Function  TreatAsAtomicUnit=on
  wires:
  Constant/1 -> reset_plot/1(gates)

== system Bebop10_from_exp/Navigation ==
  current spline : Inport
  std dev : Inport  Port=2
  In Bus Element : Inport  Port=3  PortName=WP_all  Element=list
  In Bus Element3 : Inport  Port=3  PortName=WP_all  Element=idx
  In Bus Element1 : Inport  Port=4  PortName=state  Element=pos
  auto : Inport  Port=5
  Constant : Constant  Value=two_std_dev_thres
  Scope : Scope  NumInputPorts=5
  Terminator : Terminator
  calc v : Subsystem
  calculate desired : Subsystem
  get WPts : Subsystem
  select d : MATLAB Function  TreatAsAtomicUnit=on
  set position : Subsystem
  Bus Element Out : Outport  PortName=SP_des  Element=pos
  Bus Element Out1 : Outport  PortName=SP_des  Element=vel
  Bus Element Out2 : Outport  PortName=SP_des  Element=yaw
  d new raw : Outport  Port=2
  wires:
  calculate desired/2(WP vel des) -> Bus Element Out1/1
  current spline/1 -> calc v/1(current spline), calculate desired/2(current spline), set position/1(current spline)
  calculate desired/1(yaw) -> Bus Element Out2/1
  In Bus Element1/1 -> calculate desired/5(drone current pos), calc v/3(drone current pos)
  set position/2(d new raw) -> d new raw/1
  get WPts/3(WP next) -> calculate desired/7(WP next)
  get WPts/2(WP this) -> calc v/4(WP this), calculate desired/6(WP this)
  std dev/1 -> select d/2(std_dev), calculate desired/1(std dev), calc v/2(std dev)
  set position/1(d old1) -> Scope/4, select d/1("d_old "), calculate desired/3(d)
  calculate desired/3(pos) -> calc v/5(drone desired pos), Bus Element Out/1
  calc v/1(velocity) -> Scope/2, calculate desired/4(vel), set position/2(velocity)
  In Bus Element/1 -> get WPts/1(list)
  In Bus Element3/1 -> get WPts/2(idx)
  select d/1(d_old) -> set position/3(d old), calc v/6(d)
  get WPts/1(WP last) -> Terminator/1
  auto/1 -> set position/4(auto)
  Constant/1 -> select d/3(two_std_dev_thres)

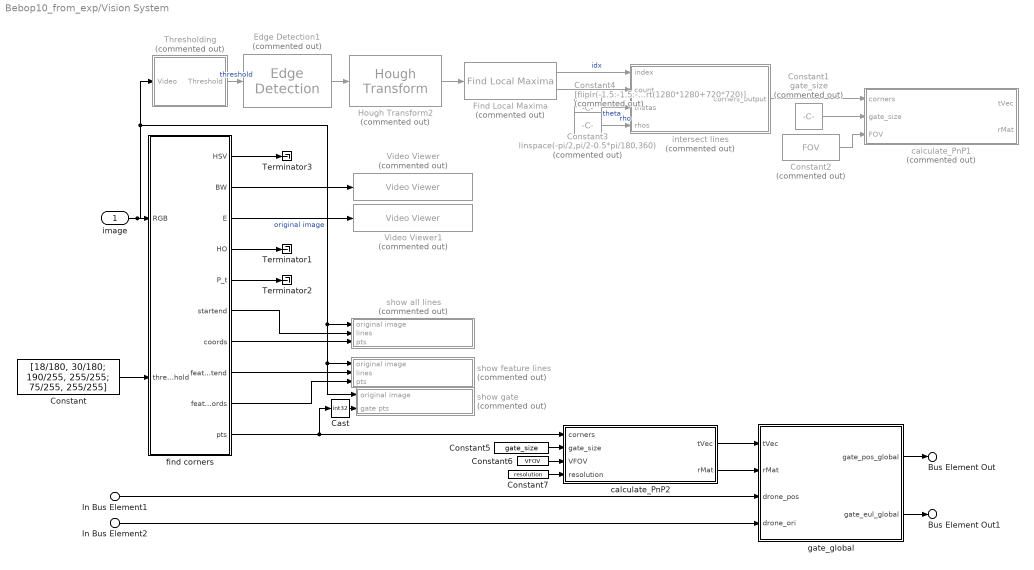
== system Bebop10_from_exp/Vision System ==
  image : Inport
  In Bus Element1 : Inport  Port=2  PortName=state  Element=pos
  In Bus Element2 : Inport  Port=2  PortName=state  Element=eul
  Cast : DataTypeConversion  OutDataTypeStr=int32
  Constant : Constant  Value=[18/180, 30/180; 190/255, 255/255; 75/255, 255/255]  VectorParams1D=off
  Constant1 : Constant  Commented=on  Value=gate_size
  Constant2 : Constant  Commented=on  Value=FOV
  Constant3 : Constant  Commented=on  Value=linspace(-pi/2,pi/2-0.5*pi/180,360)
  Constant4 : Constant  Commented=on  Value=[fliplr(-1.5:-1.5:-sqrt(1280*1280+720*720)), 0:1.5:sqrt(1280*1280+720*720)]
  Constant5 : Constant  Value=gate_size
  Constant6 : Constant  Value=VFOV
  Constant7 : Constant  Value=resolution  VectorParams1D=off
  Edge Detection1 : visionanalysis/Edge Detection  Commented=on  method=Sobel  outputType=Binary image  userDefinedThreshold=off  thresholdSource=Input port  threshold=20  thresholdTuning=20  edgeThinning=on  threshold_canny=[0.25 0.60]  autoPercent=70  sigma=1  roundingMode=Floor  overflowMode=off  prodOutputMode=Binary point scaling  prodOutputWordLength=32  prodOutputFracLength=8  prodOutputSlope=2^-8  accumSlope=2^-8  outputSlope=2^-4
      settings: SourceProductName=Computer Vision System Toolbox  SourceProductBaseCode=VP
  Find Local Maxima : visionstatistics/Find Local Maxima  Commented=on  num_peaks=8  nhood_size=[7 15]  src_thresh=Obsolete9b  src_thresh_inuse=Specify via dialog  threshold=100  inputIsHough=on  dt_peak=uint32  isOutVarDim=off  dt_count=uint32
      settings: SourceProductName=Computer Vision System Toolbox  SourceProductBaseCode=VP
  Hough Transform2 : visiontransforms/Hough Transform  Commented=on  theta_res=0.5*pi/180  rho_res=1.5  out_theta_rho=off  outdtmode=double  firstCoeffMode=Binary point scaling  firstCoeffWordLength=16  firstCoeffFracLength=14  secondCoeffMode=Binary point scaling  secondCoeffWordLength=32  secondCoeffFracLength=16  outputMode=Binary point scaling  outputWordLength=16  outputFracLength=0  accumMode=Binary point scaling  accumWordLength=32  accumFracLength=20  prodOutputMode=Binary point scaling  prodOutputWordLength=32  prodOutputFracLength=20  memoryMode=Binary point scaling  memoryWordLength=32  memoryFracLength=16  roundingMode=Nearest  overflowMode=on
      settings: SourceProductName=Computer Vision System Toolbox  SourceProductBaseCode=VP
  Terminator1 : Terminator
  Terminator2 : Terminator
  Terminator3 : Terminator
  Thresholding : Subsystem  Commented=on
  Video Viewer : VideoViewer  Commented=on  colormapValue=gray(256)  FigPos=[574 1078 1347 945]
  Video Viewer1 : VideoViewer  Commented=on  colormapValue=gray(256)  FigPos=[575 1078 1346 945]
  calculate_PnP1 : MATLAB Function  Commented=on  TreatAsAtomicUnit=on
  calculate_PnP2 : MATLAB Function  TreatAsAtomicUnit=on
  find corners : MATLAB Function  TreatAsAtomicUnit=on
  gate_global : MATLAB Function  TreatAsAtomicUnit=on
  intersect lines : MATLAB Function  Commented=on  TreatAsAtomicUnit=on
  show all lines : Subsystem  Commented=on
  show feature lines : Subsystem  Commented=on
  show gate : Subsystem  Commented=on
  Bus Element Out : Outport  PortName=WP_curr  Element=pos
  Bus Element Out1 : Outport  PortName=WP_curr  Element=eul
  wires:
  Find Local Maxima/1 -> intersect lines/1(index)  "idx"
  Edge Detection1/1 -> Hough Transform2/1
  Constant3/1 -> intersect lines/3(thetas)  "theta"
  Constant4/1 -> intersect lines/4(rhos)  "rho"
  image/1 -> show gate/1(original image), show feature lines/1(original image), show all lines/1(original image), Thresholding/1("Video "), find corners/1(RGB)  "original image"
  Constant1/1 -> calculate_PnP1/2(gate_size)
  Constant2/1 -> calculate_PnP1/3(FOV)
  In Bus Element2/1 -> gate_global/4(drone_ori)
  In Bus Element1/1 -> gate_global/3(drone_pos)
  gate_global/2(gate_eul_global) -> Bus Element Out1/1
  gate_global/1(gate_pos_global) -> Bus Element Out/1
  Hough Transform2/1 -> Find Local Maxima/1
  Find Local Maxima/2 -> intersect lines/2(count)
  intersect lines/1(corners_output) -> calculate_PnP1/1(corners)
  Thresholding/1(Threshold) -> Edge Detection1/1  "threshold"
  Constant6/1 -> calculate_PnP2/3(VFOV)
  Constant5/1 -> calculate_PnP2/2(gate_size)
  calculate_PnP2/1(tVec) -> gate_global/1(tVec)
  calculate_PnP2/2(rMat) -> gate_global/2(rMat)
  find corners/8(features_startend) -> show feature lines/2(lines)
  find corners/9(features_coords) -> show feature lines/3(pts)
  find corners/6(startend) -> show all lines/2(lines)
  find corners/7(coords) -> show all lines/3(pts)
  find corners/5(P_t) -> Terminator2/1
  find corners/4(HO) -> Terminator1/1
  find corners/3(E) -> Video Viewer1/1
  find corners/10(pts) -> Cast/1, calculate_PnP2/1(corners)
  Cast/1 -> show gate/2(gate pts)
  find corners/2(BW) -> Video Viewer/1
  Constant/1 -> find corners/2(threshold)
  find corners/1(HSV) -> Terminator3/1
  Constant7/1 -> calculate_PnP2/4(resolution)

== system Bebop10_from_exp/conv ==
  In Bus Element : Inport  PortName=state  Element=eul
  In Bus Element1 : Inport  PortName=state  Element=pos
  global2strange drone : Subsystem
  axang : Outport
  pos : Outport  Port=2
  wires:
  In Bus Element/1 -> global2strange drone/1(euler global)
  global2strange drone/1(axang strange) -> axang/1
  In Bus Element1/1 -> pos/1

== system Bebop10_from_exp/Bebop model/Rotation Controller ==
  R Des : Inport
  R Curr : Inport  Port=2
  Gain : Gain  Gain=I(3,3)
  PID Controller : simulink/Continuous/PID Controller  Controller=PID  TimeDomain=Continuous-time  SampleTime=-1  IntegratorMethod=Forward Euler  FilterMethod=Forward Euler  Form=Parallel  UseFilter=on  ControllerParametersSource=internal  P=10  I=.3  D=.1  N=100  InitialConditionSource=internal  InitialConditionForIntegrator=0  InitialConditionForFilter=0  ExternalReset=none  LimitOutput=off  UpperSaturationLimit=inf  LowerSaturationLimit=-inf  LinearizeAsGain=on  AntiWindupMode=none  Kb=1  TrackingMode=off  Kt=1  PParamMin=[]  PParamMax=[]  IParamMin=[]  IParamMax=[]  DParamMin=[]  DParamMax=[]  NParamMin=[]  NParamMax=[]  KbParamMin=[]  KbParamMax=[]  KtParamMin=[]  KtParamMax=[]  POutMin=[]  POutMax=[]  IOutMin=[]  IOutMax=[]  DOutMin=[]  DOutMax=[]  NOutMin=[]  NOutMax=[]  KbOutMin=[]  KbOutMax=[]  KtOutMin=[]  KtOutMax=[]  IntegratorOutMin=[]  IntegratorOutMax=[]  FilterOutMin=[]  FilterOutMax=[]  SumOutMin=[]  SumOutMax=[]  SumI1OutMin=[]  SumI1OutMax=[]  SumI2OutMin=[]  SumI2OutMax=[]  SumI3OutMin=[]  SumI3OutMax=[]  SumDOutMin=[]  SumDOutMax=[]  SaturationOutMin=[]  SaturationOutMax=[]  IntegratorContinuousStateAttributes=''  IntegratorStateMustResolveToSignalObject=off  IntegratorRTWStateStorageClass=Auto  FilterContinuousStateAttributes=''  FilterStateMustResolveToSignalObject=off  FilterRTWStateStorageClass=Auto  DifferentiatorICPrevScaledInput=0  DifferentiatorOutMin=[]  DifferentiatorOutMax=[]  FilterDiffOutCoefMin=[]  FilterDiffOutCoefMax=[]  SumDenOutMin=[]  SumDenOutMax=[]  SumNumOutMin=[]  SumNumOutMax=[]  ReciprocalOutMin=[]  ReciprocalOutMax=[]  DivideOutMin=[]  DivideOutMax=[]  TunerSelectOption=Transfer Function Based (PID Tuner App)
  Scope : Scope  NumInputPorts=2
  Sum : Sum  Inputs=|+-
  Torque : Outport
  wires:
  R Des/1 -> Scope/1, Sum/1  "R Des"
  Sum/1 -> PID Controller/1
  R Curr/1 -> Scope/2, Sum/2  "R Curr"
  Gain/1 -> Torque/1
  PID Controller/1 -> Gain/1

== system Bebop10_from_exp/Bebop model/Z Vel Controller ==
  Z Des : Inport
  Z Curr : Inport  Port=2
  Gain : Gain  Gain=m
  PID Controller : simulink/Continuous/PID Controller  Controller=PID  TimeDomain=Continuous-time  SampleTime=-1  IntegratorMethod=Forward Euler  FilterMethod=Forward Euler  Form=Parallel  UseFilter=on  ControllerParametersSource=internal  P=5  I=.15  D=.1  N=100  InitialConditionSource=internal  InitialConditionForIntegrator=0  InitialConditionForFilter=0  ExternalReset=none  LimitOutput=off  UpperSaturationLimit=inf  LowerSaturationLimit=-inf  LinearizeAsGain=on  AntiWindupMode=none  Kb=1  TrackingMode=off  Kt=1  PParamMin=[]  PParamMax=[]  IParamMin=[]  IParamMax=[]  DParamMin=[]  DParamMax=[]  NParamMin=[]  NParamMax=[]  KbParamMin=[]  KbParamMax=[]  KtParamMin=[]  KtParamMax=[]  POutMin=[]  POutMax=[]  IOutMin=[]  IOutMax=[]  DOutMin=[]  DOutMax=[]  NOutMin=[]  NOutMax=[]  KbOutMin=[]  KbOutMax=[]  KtOutMin=[]  KtOutMax=[]  IntegratorOutMin=[]  IntegratorOutMax=[]  FilterOutMin=[]  FilterOutMax=[]  SumOutMin=[]  SumOutMax=[]  SumI1OutMin=[]  SumI1OutMax=[]  SumI2OutMin=[]  SumI2OutMax=[]  SumI3OutMin=[]  SumI3OutMax=[]  SumDOutMin=[]  SumDOutMax=[]  SaturationOutMin=[]  SaturationOutMax=[]  IntegratorContinuousStateAttributes=''  IntegratorStateMustResolveToSignalObject=off  IntegratorRTWStateStorageClass=Auto  FilterContinuousStateAttributes=''  FilterStateMustResolveToSignalObject=off  FilterRTWStateStorageClass=Auto  DifferentiatorICPrevScaledInput=0  DifferentiatorOutMin=[]  DifferentiatorOutMax=[]  FilterDiffOutCoefMin=[]  FilterDiffOutCoefMax=[]  SumDenOutMin=[]  SumDenOutMax=[]  SumNumOutMin=[]  SumNumOutMax=[]  ReciprocalOutMin=[]  ReciprocalOutMax=[]  DivideOutMin=[]  DivideOutMax=[]  TunerSelectOption=Transfer Function Based (PID Tuner App)
  Scope : Scope  NumInputPorts=2
  Sum : Sum  Inputs=|+-
  Fz : Outport
  wires:
  Z Des/1 -> Scope/1, Sum/1  "Z Des"
  Z Curr/1 -> Scope/2, Sum/2  "Z Curr"
  Sum/1 -> PID Controller/1
  Gain/1 -> Fz/1
  PID Controller/1 -> Gain/1

== system Bebop10_from_exp/Control/Create Path Frame ==
  Velocity Vector : Inport
  Invert 3x3 Matrix : aerolibutil/Invert  3x3 Matrix
  Make X Vector : Subsystem
  Make Y Vector : Subsystem
  Make Z Vector : Subsystem
  Matrix Concatenate : Concatenate  NumInputs=3  Mode=Multidimensional array  ConcatenateDimension=2
  Rotation Matrix : Outport
  wires:
  Velocity Vector/1 -> Make Z Vector/1(Velocity Vector), Make X Vector/1(Velocity Vector), Make Y Vector/1(Velocity Vector)
  Make Y Vector/1(Y Vector) -> Matrix Concatenate/2
  Make X Vector/1(X Vector) -> Matrix Concatenate/1
  Make Z Vector/1(Z Vector) -> Matrix Concatenate/3
  Matrix Concatenate/1 -> Invert 3x3 Matrix/1
  Invert 3x3 Matrix/1 -> Rotation Matrix/1

== system Bebop10_from_exp/Control/Orientation to 3D yaw rotation ==
  note: eul2rotm
  Drone yaw : Inport
  Constant1 : Constant  Value=0
  Rotation Angles to Direction Cosine Matrix : sharedtransform/Rotation Angles to Direction Cosine Matrix  rotationOrder=ZYX  aMode=aMode
      settings: SourceProductBaseCode=AE
  Vector Concatenate : Concatenate  NumInputs=3
  rot matrix : Outport
  wires:
  Constant1/1 -> Vector Concatenate/2, Vector Concatenate/3
  Vector Concatenate/1 -> Rotation Angles to Direction Cosine Matrix/1
  Drone yaw/1 -> Vector Concatenate/1  "yaw"
  Rotation Angles to Direction Cosine Matrix/1 -> rot matrix/1  "rot matrix"

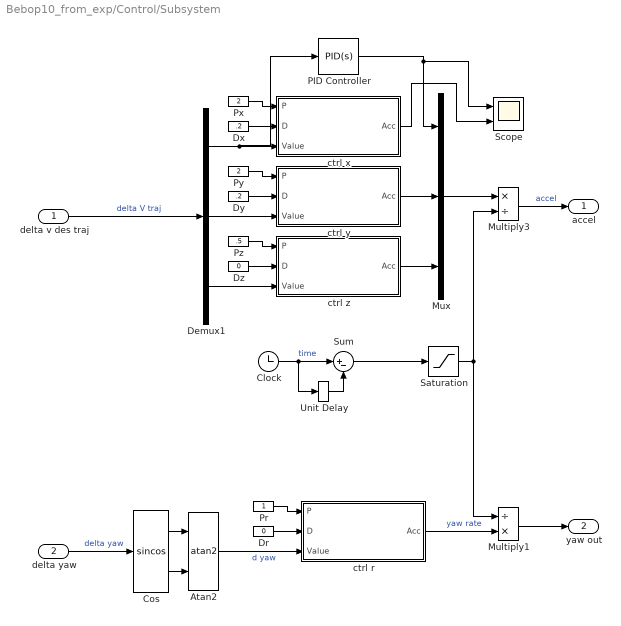
== system Bebop10_from_exp/Control/Subsystem ==
  delta v des traj : Inport
  delta yaw : Inport  Port=2
  Atan2 : Trigonometry  Operator=atan2
  Clock : Clock
  Cos : Trigonometry  Operator=sincos
  Demux1 : Demux  Outputs=3
  Dr : Constant  Value=0
  Dx : Constant  Value=.2
  Dy : Constant  Value=.2
  Dz : Constant  Value=0
  Multiply1 : Product  Inputs=/*
  Multiply3 : Product  Inputs=*/
  Mux : Mux  Inputs=3
  PID Controller : simulink/Continuous/PID Controller  Controller=PID  TimeDomain=Continuous-time  SampleTime=-1  IntegratorMethod=Forward Euler  FilterMethod=Forward Euler  Form=Parallel  UseFilter=on  ControllerParametersSource=internal  P=2  I=0  D=.2  N=100  InitialConditionSource=internal  InitialConditionForIntegrator=0  InitialConditionForFilter=0  ExternalReset=none  LimitOutput=off  UpperSaturationLimit=inf  LowerSaturationLimit=-inf  LinearizeAsGain=on  AntiWindupMode=none  Kb=1  TrackingMode=off  Kt=1  PParamMin=[]  PParamMax=[]  IParamMin=[]  IParamMax=[]  DParamMin=[]  DParamMax=[]  NParamMin=[]  NParamMax=[]  KbParamMin=[]  KbParamMax=[]  KtParamMin=[]  KtParamMax=[]  POutMin=[]  POutMax=[]  IOutMin=[]  IOutMax=[]  DOutMin=[]  DOutMax=[]  NOutMin=[]  NOutMax=[]  KbOutMin=[]  KbOutMax=[]  KtOutMin=[]  KtOutMax=[]  IntegratorOutMin=[]  IntegratorOutMax=[]  FilterOutMin=[]  FilterOutMax=[]  SumOutMin=[]  SumOutMax=[]  SumI1OutMin=[]  SumI1OutMax=[]  SumI2OutMin=[]  SumI2OutMax=[]  SumI3OutMin=[]  SumI3OutMax=[]  SumDOutMin=[]  SumDOutMax=[]  SaturationOutMin=[]  SaturationOutMax=[]  IntegratorContinuousStateAttributes=''  IntegratorStateMustResolveToSignalObject=off  IntegratorRTWStateStorageClass=Auto  FilterContinuousStateAttributes=''  FilterStateMustResolveToSignalObject=off  FilterRTWStateStorageClass=Auto  DifferentiatorICPrevScaledInput=0  DifferentiatorOutMin=[]  DifferentiatorOutMax=[]  FilterDiffOutCoefMin=[]  FilterDiffOutCoefMax=[]  SumDenOutMin=[]  SumDenOutMax=[]  SumNumOutMin=[]  SumNumOutMax=[]  ReciprocalOutMin=[]  ReciprocalOutMax=[]  DivideOutMin=[]  DivideOutMax=[]  TunerSelectOption=Transfer Function Based (PID Tuner App)
  Pr : Constant
  Px : Constant  Value=2
  Py : Constant  Value=2
  Pz : Constant  Value=.5
  Saturation : Saturate  UpperLimit=100  LowerLimit=0.00001
  Scope : Scope  NumInputPorts=2
  Sum : Sum  Inputs=|+-
  Unit Delay : UnitDelay  SampleTime=-1
  ctrl r : Subsystem
  ctrl x : Subsystem
  ctrl y : Subsystem
  ctrl z : Subsystem
  accel : Outport
  yaw out : Outport  Port=2
  wires:
  Multiply3/1 -> accel/1  "accel"
  Dz/1 -> ctrl z/2(D)
  Mux/1 -> Multiply3/1
  ctrl x/1(Acc) -> Scope/2
  Py/1 -> ctrl y/1(P)
  Dy/1 -> ctrl y/2(D)
  Unit Delay/1 -> Sum/2
  Px/1 -> ctrl x/1(P)
  ctrl y/1(Acc) -> Mux/2
  Sum/1 -> Saturation/1
  Clock/1 -> Unit Delay/1, Sum/1  "time"
  Pz/1 -> ctrl z/1(P)
  Demux1/1 -> PID Controller/1, ctrl x/3(Value)
  Dx/1 -> ctrl x/2(D)
  Demux1/2 -> ctrl y/3(Value)
  ctrl z/1(Acc) -> Mux/3
  Saturation/1 -> Multiply1/1, Multiply3/2
  Demux1/3 -> ctrl z/3(Value)
  delta v des traj/1 -> Demux1/1  "delta V traj"
  Atan2/1 -> ctrl r/3(Value)  "d yaw"
  Cos/2 -> Atan2/2
  ctrl r/1(Acc) -> Multiply1/2  "yaw rate"
  Cos/1 -> Atan2/1
  delta yaw/1 -> Cos/1  "delta yaw"
  Multiply1/1 -> yaw out/1
  Dr/1 -> ctrl r/2(D)
  Pr/1 -> ctrl r/1(P)
  PID Controller/1 -> Scope/1, Mux/1

== system Bebop10_from_exp/Gate info/Yaw2Axang1 ==
  Yaw : Inport
  Constant6 : Constant  Value=0
  Constant7 : Constant  Value=-pi/2
  Rotation Angles to Quaternions : sharedtransform/Rotation Angles to Quaternions  rotationOrder=ZYX  aMode=aMode
      settings: SourceProductName=Aerospace Blockset  SourceProductBaseCode=AE
  Subsystem : Subsystem
  Sum : Sum  Inputs=++|
  Vector Concatenate2 : Concatenate  NumInputs=3
  axang : Outport
  wires:
  Sum/1 -> Vector Concatenate2/1
  Constant7/1 -> Sum/1
  Vector Concatenate2/1 -> Rotation Angles to Quaternions/1
  Subsystem/1(Out1) -> axang/1
  Rotation Angles to Quaternions/1 -> Subsystem/1(In1)
  Constant6/1 -> Vector Concatenate2/2, Vector Concatenate2/3
  Yaw/1 -> Sum/2

== system Bebop10_from_exp/Gate info/Yaw2Axang2 ==
  Yaw : Inport
  Constant6 : Constant  Value=0
  Constant7 : Constant  Value=-pi/2
  Rotation Angles to Quaternions : sharedtransform/Rotation Angles to Quaternions  rotationOrder=ZYX  aMode=aMode
      settings: SourceProductName=Aerospace Blockset  SourceProductBaseCode=AE
  Subsystem : Subsystem
  Sum : Sum  Inputs=++|
  Vector Concatenate2 : Concatenate  NumInputs=3
  axang : Outport
  wires:
  Sum/1 -> Vector Concatenate2/1
  Constant7/1 -> Sum/1
  Vector Concatenate2/1 -> Rotation Angles to Quaternions/1
  Subsystem/1(Out1) -> axang/1
  Rotation Angles to Quaternions/1 -> Subsystem/1(In1)
  Constant6/1 -> Vector Concatenate2/2, Vector Concatenate2/3
  Yaw/1 -> Sum/2

== system Bebop10_from_exp/Gate info/Yaw2Axang3 ==
  Yaw : Inport
  Constant6 : Constant  Value=0
  Constant7 : Constant  Value=-pi/2
  Rotation Angles to Quaternions : sharedtransform/Rotation Angles to Quaternions  rotationOrder=ZYX  aMode=aMode
      settings: SourceProductName=Aerospace Blockset  SourceProductBaseCode=AE
  Subsystem : Subsystem
  Sum : Sum  Inputs=++|
  Vector Concatenate2 : Concatenate  NumInputs=3
  axang : Outport
  wires:
  Sum/1 -> Vector Concatenate2/1
  Constant7/1 -> Sum/1
  Vector Concatenate2/1 -> Rotation Angles to Quaternions/1
  Subsystem/1(Out1) -> axang/1
  Rotation Angles to Quaternions/1 -> Subsystem/1(In1)
  Constant6/1 -> Vector Concatenate2/2, Vector Concatenate2/3
  Yaw/1 -> Sum/2

== system Bebop10_from_exp/Gate info/Yaw2Axang4 ==
  Yaw : Inport
  Constant6 : Constant  Value=0
  Constant7 : Constant  Value=-pi/2
  Rotation Angles to Quaternions : sharedtransform/Rotation Angles to Quaternions  rotationOrder=ZYX  aMode=aMode
      settings: SourceProductName=Aerospace Blockset  SourceProductBaseCode=AE
  Subsystem : Subsystem
  Sum : Sum  Inputs=++|
  Vector Concatenate2 : Concatenate  NumInputs=3
  axang : Outport
  wires:
  Sum/1 -> Vector Concatenate2/1
  Constant7/1 -> Sum/1
  Vector Concatenate2/1 -> Rotation Angles to Quaternions/1
  Subsystem/1(Out1) -> axang/1
  Rotation Angles to Quaternions/1 -> Subsystem/1(In1)
  Constant6/1 -> Vector Concatenate2/2, Vector Concatenate2/3
  Yaw/1 -> Sum/2

== system Bebop10_from_exp/Gate info/Yaw2Axang5 ==
  Yaw : Inport
  Constant6 : Constant  Value=0
  Constant7 : Constant  Value=-pi/2
  Rotation Angles to Quaternions : sharedtransform/Rotation Angles to Quaternions  rotationOrder=ZYX  aMode=aMode
      settings: SourceProductName=Aerospace Blockset  SourceProductBaseCode=AE
  Subsystem : Subsystem
  Sum : Sum  Inputs=++|
  Vector Concatenate2 : Concatenate  NumInputs=3
  axang : Outport
  wires:
  Sum/1 -> Vector Concatenate2/1
  Constant7/1 -> Sum/1
  Vector Concatenate2/1 -> Rotation Angles to Quaternions/1
  Subsystem/1(Out1) -> axang/1
  Rotation Angles to Quaternions/1 -> Subsystem/1(In1)
  Constant6/1 -> Vector Concatenate2/2, Vector Concatenate2/3
  Yaw/1 -> Sum/2

== system Bebop10_from_exp/Gate info/Yaw2Axang6 ==
  Yaw : Inport
  Constant6 : Constant  Value=0
  Constant7 : Constant  Value=-pi/2
  Rotation Angles to Quaternions : sharedtransform/Rotation Angles to Quaternions  rotationOrder=ZYX  aMode=aMode
      settings: SourceProductName=Aerospace Blockset  SourceProductBaseCode=AE
  Subsystem : Subsystem
  Sum : Sum  Inputs=++|
  Vector Concatenate2 : Concatenate  NumInputs=3
  axang : Outport
  wires:
  Sum/1 -> Vector Concatenate2/1
  Constant7/1 -> Sum/1
  Vector Concatenate2/1 -> Rotation Angles to Quaternions/1
  Subsystem/1(Out1) -> axang/1
  Rotation Angles to Quaternions/1 -> Subsystem/1(In1)
  Constant6/1 -> Vector Concatenate2/2, Vector Concatenate2/3
  Yaw/1 -> Sum/2

== system Bebop10_from_exp/Gate info/Yaw2Axang7 ==
  Yaw : Inport
  Constant6 : Constant  Value=0
  Constant7 : Constant  Value=-pi/2
  Rotation Angles to Quaternions : sharedtransform/Rotation Angles to Quaternions  rotationOrder=ZYX  aMode=aMode
      settings: SourceProductName=Aerospace Blockset  SourceProductBaseCode=AE
  Subsystem : Subsystem
  Sum : Sum  Inputs=++|
  Vector Concatenate2 : Concatenate  NumInputs=3
  axang : Outport
  wires:
  Sum/1 -> Vector Concatenate2/1
  Constant7/1 -> Sum/1
  Vector Concatenate2/1 -> Rotation Angles to Quaternions/1
  Subsystem/1(Out1) -> axang/1
  Rotation Angles to Quaternions/1 -> Subsystem/1(In1)
  Constant6/1 -> Vector Concatenate2/2, Vector Concatenate2/3
  Yaw/1 -> Sum/2
